simulink model "coeff_bank_integration_test"  (R2021b)
settings: Solver=FixedStepDiscrete  StartTime=0.0  StopTime=stop_time-1  RelTol=1e-3
undefined symbols (not defined in the file): combiner_attribs, dl_filter_attribs, input_bus, splitter_attribs, ul_filter_attribs
libraries: dspsrcs4 x20
settings Model: DataTypeOverride=Off  Creator=torha  LastModifiedBy=torha
settings OptimizationCC: BlockReduction=off  ConditionallyExecuteInputs=off  DefaultParameterBehavior=Inlined  InheritOutputTypeSmallerThanSingle=on
settings DebuggingCC: AlgebraicLoopMsg=error  SingleTaskRateTransMsg=error
settings HardwareCC: ProdBitPerPointer=32  ProdBitPerSizeT=32  ProdBitPerPtrDiffT=32  ProdLargestAtomicFloat=None  ProdIntDivRoundTo=Undefined  ProdEndianess=Unspecified  ProdWordSize=32  ProdHWDeviceType=ASIC/FPGA->ASIC/FPGA  TargetBitPerPointer=64  TargetBitPerSizeT=64  TargetBitPerPtrDiffT=64  TargetLongLongMode=on  TargetIntDivRoundTo=Zero  TargetEndianess=LittleEndian  TargetWordSize=64  TargetHWDeviceType=Custom Processor->MATLAB Host Computer  ProdEqTarget=off

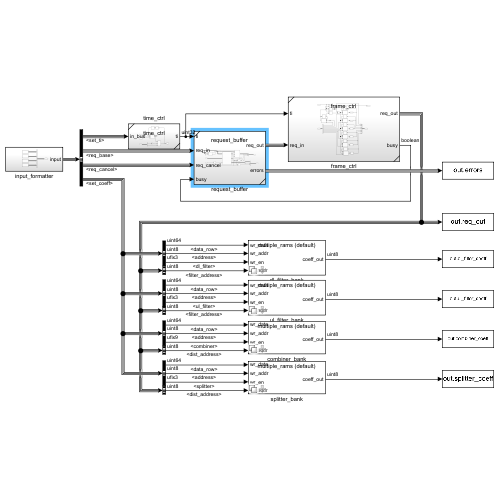
[thumbnail: Simulink's stored preview of the top-level diagram]
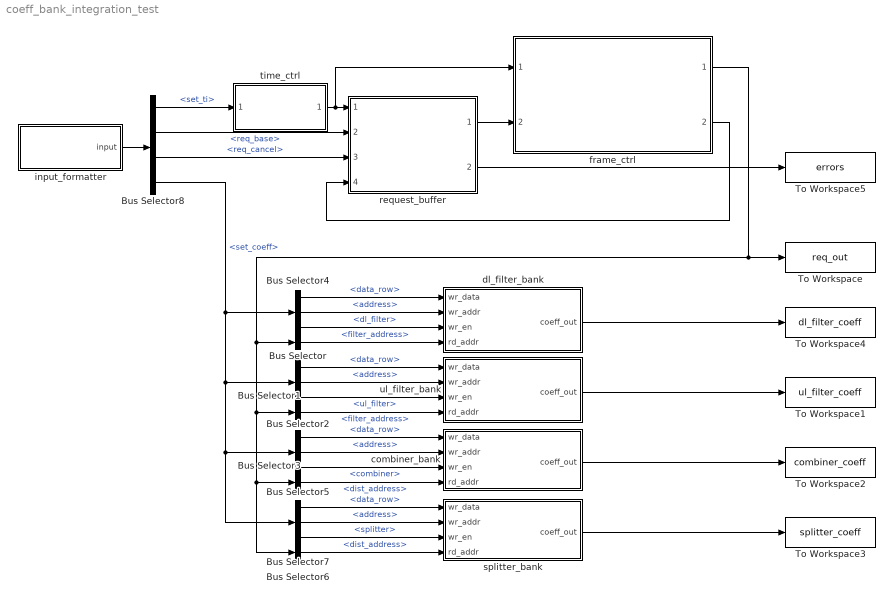
== system coeff_bank_integration_test ==
  Bus Selector : BusSelector  OutputSignals=filter_address
  Bus Selector1 : BusSelector  OutputSignals=filter_address
  Bus Selector2 : BusSelector  OutputSignals=data_row,address,ul_filter
  Bus Selector3 : BusSelector  OutputSignals=dist_address
  Bus Selector4 : BusSelector  OutputSignals=data_row,address,dl_filter
  Bus Selector5 : BusSelector  OutputSignals=data_row,address,combiner
  Bus Selector6 : BusSelector  OutputSignals=dist_address
  Bus Selector7 : BusSelector  OutputSignals=data_row,address,splitter
  Bus Selector8 : BusSelector  OutputSignals=set_ti,req_base,req_cancel,set_coeff
  To Workspace : ToWorkspace  VariableName=req_out  SaveFormat=Timeseries  SampleTime=-1
  To Workspace1 : ToWorkspace  VariableName=ul_filter_coeff  SampleTime=-1
      settings: Save2DSignal=2-D array (concatenate along first dimension)
  To Workspace2 : ToWorkspace  VariableName=combiner_coeff  SampleTime=-1
      settings: Save2DSignal=2-D array (concatenate along first dimension)
  To Workspace3 : ToWorkspace  VariableName=splitter_coeff  SampleTime=-1
      settings: Save2DSignal=2-D array (concatenate along first dimension)
  To Workspace4 : ToWorkspace  VariableName=dl_filter_coeff  SampleTime=-1
      settings: Save2DSignal=2-D array (concatenate along first dimension)
  To Workspace5 : ToWorkspace  VariableName=errors  SaveFormat=Timeseries  SampleTime=-1
  combiner_bank : Subsystem  Variant=on  mask{coeff=combiner_attribs}
      mask init:
      | load('constants.mat', 'coeff_ram_bitwidth');
      | last_ram_size = mod(coeff.coeff_bitwidth*coeff.coeff_num*(1+coeff.complex), coeff_ram_bitwidth);
      | if last_ram_size == 0
      |     last_ram_size = coeff_ram_bitwidth;
      | end
      | num_rams = ceil(coeff.coeff_bitwidth*coeff.coeff_num*(1+coeff.complex)/coeff_ram_bitwidth)-1;
  dl_filter_bank : Subsystem  Variant=on  mask{coeff=dl_filter_attribs}
      mask init: same as coeff_bank_integration_test/combiner_bank
  frame_ctrl : Subsystem  ReferencedSubsystem=frame_ctrl
  input_formatter : Subsystem
  request_buffer : Subsystem  ReferencedSubsystem=request_buffer
  splitter_bank : Subsystem  Variant=on  mask{coeff=splitter_attribs}
      mask init: same as coeff_bank_integration_test/combiner_bank
  time_ctrl : Subsystem  ReferencedSubsystem=time_ctrl
  ul_filter_bank : Subsystem  Variant=on  mask{coeff=ul_filter_attribs}
      mask init: same as coeff_bank_integration_test/combiner_bank
  wires:
  frame_ctrl/2 -> request_buffer/4
  time_ctrl/1 -> request_buffer/1, frame_ctrl/1
  Bus Selector8/1 -> time_ctrl/1  "<set_ti>"
  request_buffer/1 -> frame_ctrl/2
  Bus Selector8/3 -> request_buffer/3  "<req_cancel>"
  Bus Selector8/2 -> request_buffer/2  "<req_base>"
  dl_filter_bank/1(coeff_out) -> To Workspace4/1
  ul_filter_bank/1(coeff_out) -> To Workspace1/1
  combiner_bank/1(coeff_out) -> To Workspace2/1
  splitter_bank/1(coeff_out) -> To Workspace3/1
  Bus Selector8/4 -> Bus Selector7/1, Bus Selector5/1, Bus Selector2/1, Bus Selector4/1  "<set_coeff>"
  frame_ctrl/1 -> Bus Selector6/1, Bus Selector3/1, Bus Selector1/1, Bus Selector/1, To Workspace/1
  Bus Selector4/1 -> dl_filter_bank/1(wr_data)  "<data_row>"
  Bus Selector4/3 -> dl_filter_bank/3(wr_en)  "<dl_filter>"
  Bus Selector4/2 -> dl_filter_bank/2(wr_addr)  "<address>"
  Bus Selector/1 -> dl_filter_bank/4(rd_addr)  "<filter_address>"
  Bus Selector2/2 -> ul_filter_bank/2(wr_addr)  "<address>"
  Bus Selector2/3 -> ul_filter_bank/3(wr_en)  "<ul_filter>"
  Bus Selector2/1 -> ul_filter_bank/1(wr_data)  "<data_row>"
  Bus Selector5/1 -> combiner_bank/1(wr_data)  "<data_row>"
  Bus Selector5/3 -> combiner_bank/3(wr_en)  "<combiner>"
  Bus Selector5/2 -> combiner_bank/2(wr_addr)  "<address>"
  Bus Selector7/2 -> splitter_bank/2(wr_addr)  "<address>"
  Bus Selector7/3 -> splitter_bank/3(wr_en)  "<splitter>"
  Bus Selector7/1 -> splitter_bank/1(wr_data)  "<data_row>"
  Bus Selector1/1 -> ul_filter_bank/4(rd_addr)  "<filter_address>"
  Bus Selector3/1 -> combiner_bank/4(rd_addr)  "<dist_address>"
  Bus Selector6/1 -> splitter_bank/4(rd_addr)  "<dist_address>"
  request_buffer/2 -> To Workspace5/1
  input_formatter/1(input) -> Bus Selector8/1

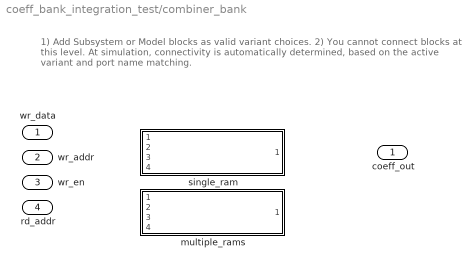
== system coeff_bank_integration_test/combiner_bank ==
  note: 1) Add Subsystem or Model blocks as valid variant choices.
      | 2) You cannot connect blocks at this level. At simulation, connectivity is automatically
      | determined, based on the active variant and port name matching.
  wr_data : Inport
  wr_addr : Inport  Port=2
  wr_en : Inport  Port=3
  rd_addr : Inport  Port=4
  multiple_rams : Subsystem  VariantControl=(default)  ReferencedSubsystem=coeff_bank_multiple_rams
  single_ram : Subsystem  VariantControl=num_rams==0  ReferencedSubsystem=coeff_bank_single_ram
  coeff_out : Outport

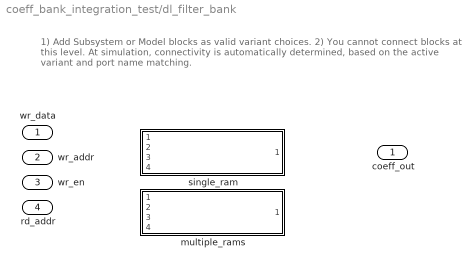
== system coeff_bank_integration_test/dl_filter_bank ==
  note: 1) Add Subsystem or Model blocks as valid variant choices.
      | 2) You cannot connect blocks at this level. At simulation, connectivity is automatically
      | determined, based on the active variant and port name matching.
  wr_data : Inport
  wr_addr : Inport  Port=2
  wr_en : Inport  Port=3
  rd_addr : Inport  Port=4
  multiple_rams : Subsystem  VariantControl=(default)  ReferencedSubsystem=coeff_bank_multiple_rams
  single_ram : Subsystem  VariantControl=num_rams==0  ReferencedSubsystem=coeff_bank_single_ram
  coeff_out : Outport

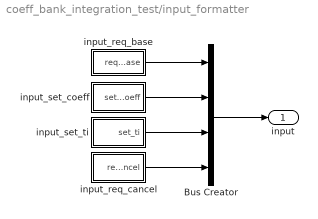
== system coeff_bank_integration_test/input_formatter ==
  Bus Creator : BusCreator  Inputs=4
  input_req_base : Subsystem
  input_req_cancel : Subsystem
  input_set_coeff : Subsystem
  input_set_ti : Subsystem
  input : Outport
  wires:
  input_req_cancel/1(req_cancel) -> Bus Creator/4
  input_set_ti/1(set_ti) -> Bus Creator/3
  input_set_coeff/1(set_coeff) -> Bus Creator/2
  input_req_base/1(req_base) -> Bus Creator/1
  Bus Creator/1 -> input/1

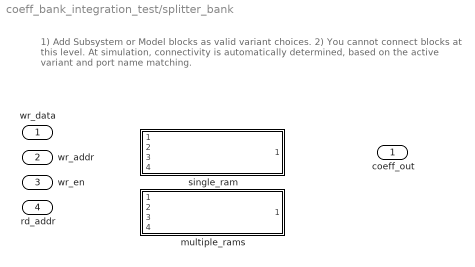
== system coeff_bank_integration_test/splitter_bank ==
  note: 1) Add Subsystem or Model blocks as valid variant choices.
      | 2) You cannot connect blocks at this level. At simulation, connectivity is automatically
      | determined, based on the active variant and port name matching.
  wr_data : Inport
  wr_addr : Inport  Port=2
  wr_en : Inport  Port=3
  rd_addr : Inport  Port=4
  multiple_rams : Subsystem  VariantControl=(default)  ReferencedSubsystem=coeff_bank_multiple_rams
  single_ram : Subsystem  VariantControl=num_rams==0  ReferencedSubsystem=coeff_bank_single_ram
  coeff_out : Outport

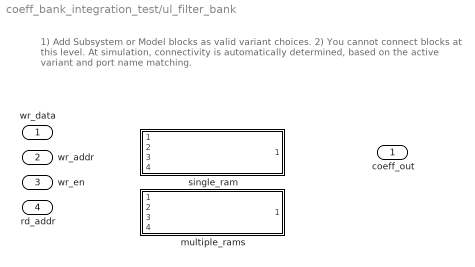
== system coeff_bank_integration_test/ul_filter_bank ==
  note: 1) Add Subsystem or Model blocks as valid variant choices.
      | 2) You cannot connect blocks at this level. At simulation, connectivity is automatically
      | determined, based on the active variant and port name matching.
  wr_data : Inport
  wr_addr : Inport  Port=2
  wr_en : Inport  Port=3
  rd_addr : Inport  Port=4
  multiple_rams : Subsystem  VariantControl=(default)  ReferencedSubsystem=coeff_bank_multiple_rams
  single_ram : Subsystem  VariantControl=num_rams==0  ReferencedSubsystem=coeff_bank_single_ram
  coeff_out : Outport

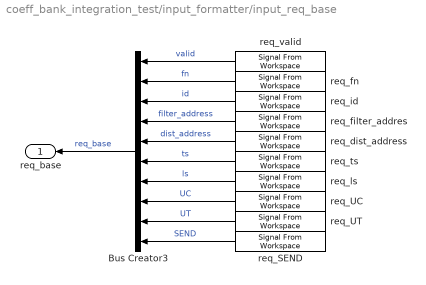
== system coeff_bank_integration_test/input_formatter/input_req_base ==
  Bus Creator3 : BusCreator  Inputs=10
  req_SEND : dspsrcs4/Signal From Workspace  X=[horzcat([input_bus.req_base]).SEND].'  Ts=1  nsamps=1  OutputAfterFinalValue=Setting to zero  ignoreOrWarnInputAndFrameLengths=off  OutputFrames=off
  req_UC : dspsrcs4/Signal From Workspace  X=[horzcat([input_bus.req_base]).UC].'  Ts=1  nsamps=1  OutputAfterFinalValue=Setting to zero  ignoreOrWarnInputAndFrameLengths=off  OutputFrames=off
  req_UT : dspsrcs4/Signal From Workspace  X=[horzcat([input_bus.req_base]).UT].'  Ts=1  nsamps=1  OutputAfterFinalValue=Setting to zero  ignoreOrWarnInputAndFrameLengths=off  OutputFrames=off
  req_dist_address : dspsrcs4/Signal From Workspace  X=[horzcat([input_bus.req_base]).dist_address].'  Ts=1  nsamps=1  OutputAfterFinalValue=Setting to zero  ignoreOrWarnInputAndFrameLengths=off  OutputFrames=off
  req_filter_addres : dspsrcs4/Signal From Workspace  X=[horzcat([input_bus.req_base]).filter_address].'  Ts=1  nsamps=1  OutputAfterFinalValue=Setting to zero  ignoreOrWarnInputAndFrameLengths=off  OutputFrames=off
  req_fn : dspsrcs4/Signal From Workspace  X=[horzcat([input_bus.req_base]).fn].'  Ts=1  nsamps=1  OutputAfterFinalValue=Setting to zero  ignoreOrWarnInputAndFrameLengths=off  OutputFrames=off
  req_id : dspsrcs4/Signal From Workspace  X=[horzcat([input_bus.req_base]).id].'  Ts=1  nsamps=1  OutputAfterFinalValue=Setting to zero  ignoreOrWarnInputAndFrameLengths=off  OutputFrames=off
  req_ls : dspsrcs4/Signal From Workspace  X=[horzcat([input_bus.req_base]).ls].'  Ts=1  nsamps=1  OutputAfterFinalValue=Setting to zero  ignoreOrWarnInputAndFrameLengths=off  OutputFrames=off
  req_ts : dspsrcs4/Signal From Workspace  X=[horzcat([input_bus.req_base]).ts].'  Ts=1  nsamps=1  OutputAfterFinalValue=Setting to zero  ignoreOrWarnInputAndFrameLengths=off  OutputFrames=off
  req_valid : dspsrcs4/Signal From Workspace  X=[horzcat([input_bus.req_base]).valid].'  Ts=1  nsamps=1  OutputAfterFinalValue=Setting to zero  ignoreOrWarnInputAndFrameLengths=off  OutputFrames=off
  req_base : Outport
  wires:
  req_UC/1 -> Bus Creator3/8  "UC"
  req_filter_addres/1 -> Bus Creator3/4  "filter_address"
  req_dist_address/1 -> Bus Creator3/5  "dist_address"
  req_fn/1 -> Bus Creator3/2  "fn"
  req_UT/1 -> Bus Creator3/9  "UT"
  req_SEND/1 -> Bus Creator3/10  "SEND"
  req_valid/1 -> Bus Creator3/1  "valid"
  req_ls/1 -> Bus Creator3/7  "ls"
  req_id/1 -> Bus Creator3/3  "id"
  req_ts/1 -> Bus Creator3/6  "ts"
  Bus Creator3/1 -> req_base/1  "req_base"

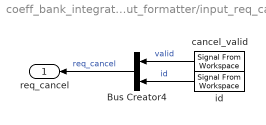
== system coeff_bank_integration_test/input_formatter/input_req_cancel ==
  Bus Creator4 : BusCreator  Inputs=2
  cancel_valid : dspsrcs4/Signal From Workspace  X=[horzcat([input_bus.req_cancel]).valid].'  Ts=1  nsamps=1  OutputAfterFinalValue=Setting to zero  ignoreOrWarnInputAndFrameLengths=off  OutputFrames=off
  id : dspsrcs4/Signal From Workspace  X=[horzcat([input_bus.req_cancel]).id].'  Ts=1  nsamps=1  OutputAfterFinalValue=Setting to zero  ignoreOrWarnInputAndFrameLengths=off  OutputFrames=off
  req_cancel : Outport
  wires:
  id/1 -> Bus Creator4/2  "id"
  cancel_valid/1 -> Bus Creator4/1  "valid"
  Bus Creator4/1 -> req_cancel/1  "req_cancel"

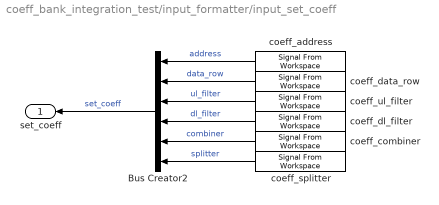
== system coeff_bank_integration_test/input_formatter/input_set_coeff ==
  Bus Creator2 : BusCreator  Inputs=6
  coeff_address : dspsrcs4/Signal From Workspace  X=[horzcat([input_bus.set_coeff]).address].'  Ts=1  nsamps=1  OutputAfterFinalValue=Setting to zero  ignoreOrWarnInputAndFrameLengths=off  OutputFrames=off
  coeff_combiner : dspsrcs4/Signal From Workspace  X=[horzcat([input_bus.set_coeff]).combiner].'  Ts=1  nsamps=1  OutputAfterFinalValue=Setting to zero  ignoreOrWarnInputAndFrameLengths=off  OutputFrames=off
  coeff_data_row : dspsrcs4/Signal From Workspace  X=[horzcat([input_bus.set_coeff]).data_row].'  Ts=1  nsamps=1  OutputAfterFinalValue=Setting to zero  ignoreOrWarnInputAndFrameLengths=off  OutputFrames=off
  coeff_dl_filter : dspsrcs4/Signal From Workspace  X=[horzcat([input_bus.set_coeff]).dl_filter].'  Ts=1  nsamps=1  OutputAfterFinalValue=Setting to zero  ignoreOrWarnInputAndFrameLengths=off  OutputFrames=off
  coeff_splitter : dspsrcs4/Signal From Workspace  X=[horzcat([input_bus.set_coeff]).splitter].'  Ts=1  nsamps=1  OutputAfterFinalValue=Setting to zero  ignoreOrWarnInputAndFrameLengths=off  OutputFrames=off
  coeff_ul_filter : dspsrcs4/Signal From Workspace  X=[horzcat([input_bus.set_coeff]).ul_filter].'  Ts=1  nsamps=1  OutputAfterFinalValue=Setting to zero  ignoreOrWarnInputAndFrameLengths=off  OutputFrames=off
  set_coeff : Outport
  wires:
  coeff_ul_filter/1 -> Bus Creator2/3  "ul_filter"
  coeff_dl_filter/1 -> Bus Creator2/4  "dl_filter"
  coeff_address/1 -> Bus Creator2/1  "address"
  coeff_splitter/1 -> Bus Creator2/6  "splitter"
  coeff_data_row/1 -> Bus Creator2/2  "data_row"
  coeff_combiner/1 -> Bus Creator2/5  "combiner"
  Bus Creator2/1 -> set_coeff/1  "set_coeff"

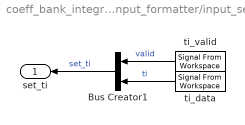
== system coeff_bank_integration_test/input_formatter/input_set_ti ==
  Bus Creator1 : BusCreator  Inputs=2
  ti_data : dspsrcs4/Signal From Workspace  X=[horzcat([input_bus.set_ti]).ti].'  Ts=1  nsamps=1  OutputAfterFinalValue=Setting to zero  ignoreOrWarnInputAndFrameLengths=off  OutputFrames=off
  ti_valid : dspsrcs4/Signal From Workspace  X=[horzcat([input_bus.set_ti]).valid].'  Ts=1  nsamps=1  OutputAfterFinalValue=Setting to zero  ignoreOrWarnInputAndFrameLengths=off  OutputFrames=off
  set_ti : Outport
  wires:
  ti_valid/1 -> Bus Creator1/1  "valid"
  ti_data/1 -> Bus Creator1/2  "ti"
  Bus Creator1/1 -> set_ti/1  "set_ti"
